simulink model "mavsim_HW3_2"  (R2016b)
settings: Solver=ode45  StartTime=0.0  StopTime=10  RelTol=1e-3
InitFcn:
  | param
undefined symbols (not defined in the file or in its folder): airdata, drawAircraft, forces_moments, P, plotmavstatevariables
libraries: simulink x4
settings Model: Creator=beard  LastModifiedBy=holly
settings DataIOCC: LimitDataPoints=on  SaveFormat=Array
settings OptimizationCC: BlockReduction=off  BooleanDataType=off  LifeSpan=inf
settings DebuggingCC: SaveWithParameterizedLinksMsg=none  UnderspecifiedInitializationDetection=Classic  MergeDetectMultiDrivingBlocksExec=none  SignalResolutionControl=TryResolveAllWithWarning  SFUnexpectedBacktrackingDiag=warning  SFNoUnconditionalDefaultTransitionDiag=warning  SFExecutionAtInitializationDiag=none
settings HardwareCC: ProdBitPerPointer=32  ProdBitPerSizeT=32  ProdBitPerPtrDiffT=32  ProdLargestAtomicFloat=None  ProdIntDivRoundTo=Undefined  ProdEndianess=Unspecified  ProdWordSize=32  ProdHWDeviceType=32-bit Generic  TargetUnknown=on
settings ModelReferenceCC: PropagateSignalLabelsOutOfModel=off
settings GRTTargetCC: TargetLangStandard=C89/C90 (ANSI)  GeneratePreprocessorConditionals=Disable all
settings ConfigComp: CovMetricSettings=dw  CovHtmlReporting=on  CovSaveCumulativeToWorkspaceVar=on  CovSaveSingleToWorkspaceVar=on  CovExternalEMLEnable=off  CovSFcnEnable=off

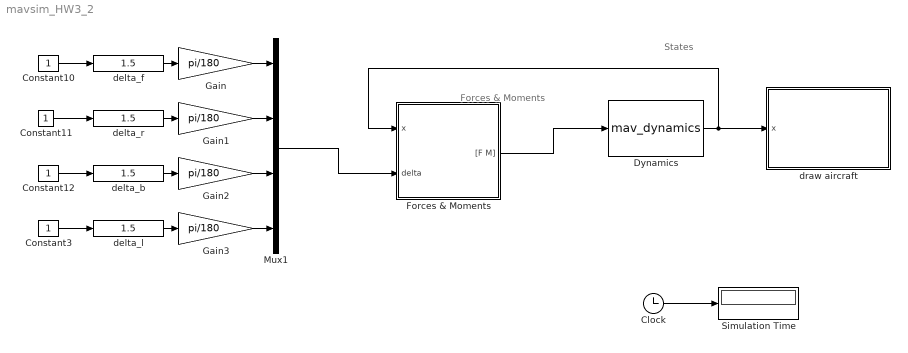
== system mavsim_HW3_2 ==
  note: Forces & Moments
  note: States
  Clock : Clock
  Constant{3,10..12} (4 alike) : Constant
  Dynamics : S-Function  FunctionName=mav_dynamics  Parameters=P  SFunctionDeploymentMode=off  EnableBusSupport=off
  Forces & Moments : Subsystem
  Gain{,1..3} (4 alike) : Gain  Gain=pi/180
  Mux1 : Mux
  Simulation Time : Display
  delta_b : simulink/Math Operations/Slider Gain  low=-20  gain=1.5  high=20
  delta_f : simulink/Math Operations/Slider Gain  low=-20  gain=1.5  high=20
  delta_l : simulink/Math Operations/Slider Gain  low=-20  gain=1.5  high=20
  delta_r : simulink/Math Operations/Slider Gain  low=-20  gain=1.5  high=20
  draw aircraft : Subsystem
      mask Display: image(imread('predator.jpg'))
  wires:
  Constant10/1 -> delta_f/1
  Constant11/1 -> delta_r/1
  Constant12/1 -> delta_b/1
  Dynamics/1 -> draw aircraft/1(x), Forces & Moments/1(x)
  delta_b/1 -> Gain2/1
  delta_r/1 -> Gain1/1
  delta_f/1 -> Gain/1
  Constant3/1 -> delta_l/1
  Mux1/1 -> Forces & Moments/2(delta)
  Forces & Moments/1("[F M]") -> Dynamics/1
  Clock/1 -> Simulation Time/1
  Gain/1 -> Mux1/1
  Gain1/1 -> Mux1/2
  Gain2/1 -> Mux1/3
  delta_l/1 -> Gain3/1
  Gain3/1 -> Mux1/4

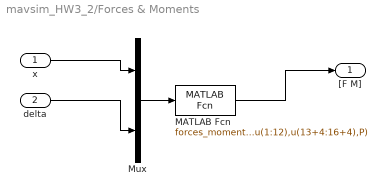
== system mavsim_HW3_2/Forces & Moments ==
  x : Inport
  delta : Inport  Port=2
  MATLAB Fcn : MATLABFcn  MATLABFcn=forces_moments(u(1:12),u(13+4:16+4),P)  OutputDimensions=6
  Mux : Mux  Inputs=2
  "[F M]" : Outport
  wires:
  x/1 -> Mux/1
  delta/1 -> Mux/2
  Mux/1 -> MATLAB Fcn/1
  MATLAB Fcn/1 -> "[F M]"/1

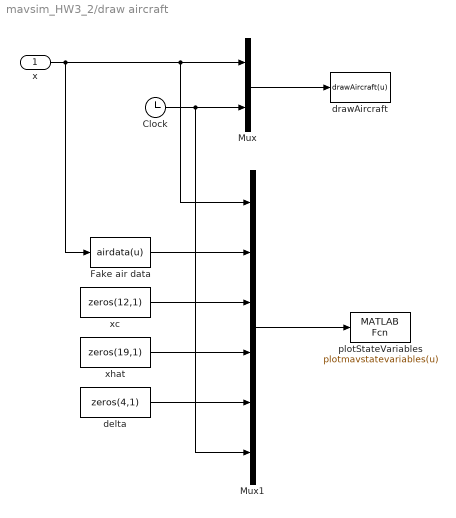
== system mavsim_HW3_2/draw aircraft ==
  x : Inport
  Clock : Clock
  Fake air data : MATLABFcn  MATLABFcn=airdata(u)  OutputDimensions=6  SampleTime=0.1
  Mux : Mux  Inputs=2
  Mux1 : Mux  Inputs=6
  delta : Constant  Value=zeros(4,1)
  drawAircraft : MATLABFcn  MATLABFcn=drawAircraft(u)  OutputDimensions=0  SampleTime=0.1
  plotStateVariables : MATLABFcn  MATLABFcn=plotmavstatevariables(u)  OutputDimensions=0  SampleTime=0.1
  xc : Constant  Value=zeros(12,1)
  xhat : Constant  Value=zeros(19,1)
  wires:
  Fake air data/1 -> Mux1/2
  delta/1 -> Mux1/5
  xc/1 -> Mux1/3
  xhat/1 -> Mux1/4
  Mux1/1 -> plotStateVariables/1
  Clock/1 -> Mux1/6, Mux/2
  x/1 -> Fake air data/1, Mux1/1, Mux/1
  Mux/1 -> drawAircraft/1
